simulink model "Modeloplanta"  (R2019a)
settings: Solver=VariableStepAuto  StartTime=0.0  StopTime=10.0  RelTol=1e-3
values from neighbouring files (symbols this model uses):
  A = 2.7    [parámetros.m]
  B = 0.1    [parámetros.m]
  Cr = 0.9    [parámetros.m]
  g = 9.81    [parámetros.m]
  J = 0.002    [parámetros.m]
  K = 0.21    [parámetros.m]
  k = 6.1e-3    (= 0.0061)    [parámetros.m]
  K_bat = (72 / sqrt(3)) / Vdc    [parámetros.m]
  Ki = 7e-1    (= 0.7)    [parámetros.m]
  Kin = 0.6 * (Vdc / Vcm)    [parámetros.m]
  Kp = 105.999    [parámetros.m]
  Kt = sqrt(3) * lamdaf * npp    [parámetros.m]
  L = 86e-6    (= 8.6e-05)    [parámetros.m]
  lamdaf = 0.03    [parámetros.m]
  Loss = 1e-3    (= 0.001)    [parámetros.m]
  Mt = 700    [parámetros.m]
  npp = 16    [parámetros.m]
  Q0 = 3.3 * 72    (= 237.6)    [parámetros.m]
  Qmax = 3.3 * 72    (= 237.6)    [parámetros.m]
  r = 0.049    [parámetros.m]
  rho = 1.3    [parámetros.m]
  RPM_MAX = 800    [parámetros.m]
  rr = 0.3    [parámetros.m]
  Tin = 1 / (2 * fc)    (= 6.25e-05)    [parámetros.m]
  TORQUE_MAX = 140    [parámetros.m]
  Ts = 1e-6    (= 1e-06)    [parámetros.m]
  V = Vdc    (= 106)    [parámetros.m]
  Varnoise = 0    [parámetros.m]
  Vmax = (1/sqrt(3)) * Vdc    [parámetros.m]
  Xnoise = 0    [parámetros.m]
undefined symbols (not defined in the file or in its folder): CARGA
libraries: simulink x1
settings Model: Creator=luisd  LastModifiedBy=luisd

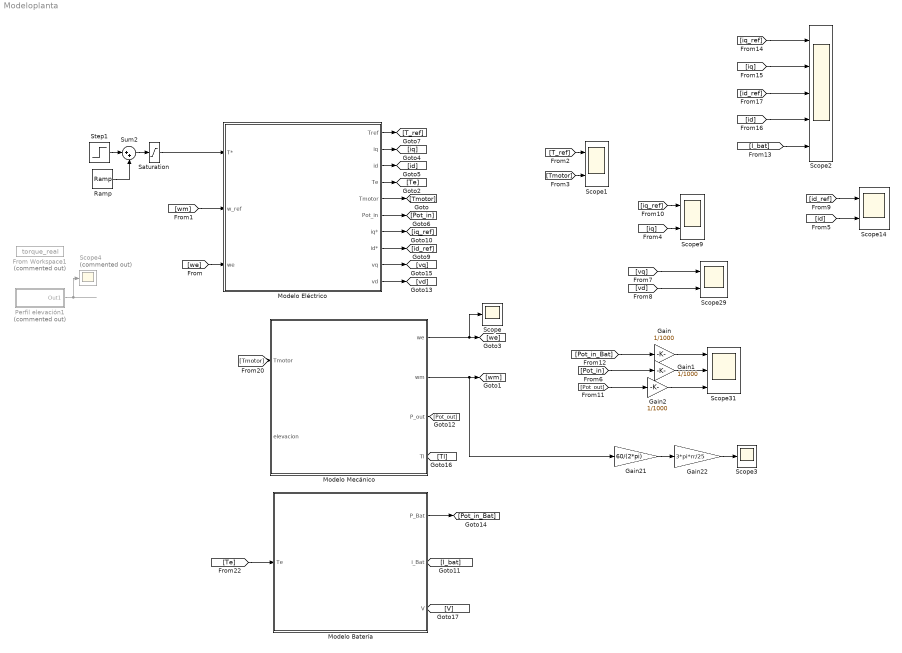
== system Modeloplanta ==
  From Workspace1 : FromWorkspace  Commented=on  VariableName=torque_real
  Gain : Gain  Gain=1/1000
  Gain1 : Gain  Gain=1/1000
  Gain2 : Gain  Gain=1/1000
  Gain21 : Gain  Gain=60/(2*pi)
  Gain22 : Gain  Gain=3*pi*rr/25
  Modelo Batería : Subsystem
  Modelo Eléctrico : Subsystem
      mask Display: image(imread('SEVCON-GEN4-SIZE-42.png'))
  Modelo Mecánico : Subsystem
      mask Display: image(imread('qs.png'))
  Perfil elevación1 : Subsystem  Commented=on
  Ramp : simulink/Sources/Ramp  slope=1e4  start=0.45  InitialOutput=0
  Saturation : Saturate  UpperLimit=5  LowerLimit=0  ZeroCross=off
  Scope : Scope
  Scope{1,9,14,29} (4 alike) : Scope  NumInputPorts=2
  Scope2 : Scope  NumInputPorts=5
  Scope3 : Scope
  Scope31 : Scope  NumInputPorts=3
  Scope4 : Scope  Commented=on
  Step1 : Step  Time=0.5  SampleTime=0
  Sum2 : Sum  Inputs=|++
  wires:
  Gain21/1 -> Gain22/1
  [id] -> Scope2/4
  [vd] -> Scope29/2
  Modelo Eléctrico/3(id) -> [id]
  [iq] -> Scope2/2
  Modelo Eléctrico/5(Tmotor) -> [Tmotor]
  Modelo Eléctrico/1(Tref) -> [T_ref]
  [id_ref] -> Scope2/3
  [I_bat] -> Scope2/5
  [wm] -> Modelo Eléctrico/2(w_ref)
  Modelo Mecánico/3(P_out) -> [Pot_out]
  Gain22/1 -> Scope3/1
  Sum2/1 -> Saturation/1
  Modelo Eléctrico/7(iq*) -> [iq_ref]
  Modelo Mecánico/1(we) -> Scope/1, [we]
  Modelo Eléctrico/8(id*) -> [id_ref]
  Modelo Mecánico/2(wm) -> Gain21/1, [wm]
  Saturation/1 -> Modelo Eléctrico/1(T*)
  [we] -> Modelo Eléctrico/3(we)
  [Pot_in_Bat] -> Gain/1
  Ramp/1 -> Sum2/2
  [vq] -> Scope29/1
  Modelo Batería/1("P_Bat ") -> [Pot_in_Bat]
  [iq_ref] -> Scope9/1
  Modelo Batería/2(i_Bat) -> [I_bat]
  [Tmotor] -> Scope1/2
  Modelo Eléctrico/9(vq) -> [vq]
  Modelo Eléctrico/2(iq) -> [iq]
  [id_ref] -> Scope14/1
  [Pot_out] -> Gain2/1
  Modelo Mecánico/4(Tl) -> [Tl]
  [Pot_in] -> Gain1/1
  Step1/1 -> Sum2/1
  Gain/1 -> Scope31/1
  Modelo Eléctrico/4(Te) -> [Te]
  [Tmotor] -> Modelo Mecánico/1(Tmotor)
  Modelo Eléctrico/10(vd) -> [vd]
  Perfil elevación1/1(Out1) -> Scope4/1
  Gain2/1 -> Scope31/3
  [Te] -> Modelo Batería/1(Te)
  [T_ref] -> Scope1/1
  Modelo Batería/3(V) -> [V]
  [id] -> Scope14/2
  Modelo Eléctrico/6(Pot_in) -> [Pot_in]
  [iq_ref] -> Scope2/1
  [iq] -> Scope9/2
  Gain1/1 -> Scope31/2

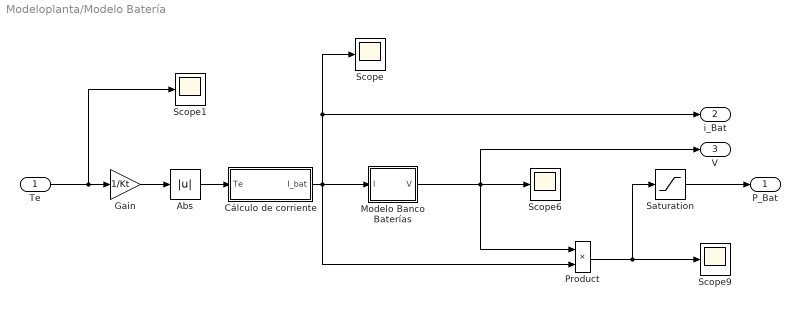
== system Modeloplanta/Modelo Batería ==
  Te : Inport
  Abs : Abs
  Cálculo de corriente : Subsystem
  Gain : Gain  Gain=1/Kt
  Modelo Banco Baterías : Subsystem
  Product : Product
  Saturation : Saturate  UpperLimit=8000  LowerLimit=-8000
  Scope{,1,6,9} (4 alike) : Scope
  "P_Bat " : Outport
  i_Bat : Outport  Port=2
  V : Outport  Port=3
  wires:
  Product/1 -> Saturation/1, Scope9/1
  Modelo Banco Baterías/1(V) -> V/1, Scope6/1, Product/1
  Cálculo de corriente/1(I_bat) -> Scope/1, i_Bat/1, Modelo Banco Baterías/1(I), Product/2
  Te/1 -> Scope1/1, Gain/1
  Saturation/1 -> "P_Bat "/1
  Gain/1 -> Abs/1
  Abs/1 -> Cálculo de corriente/1(Te)

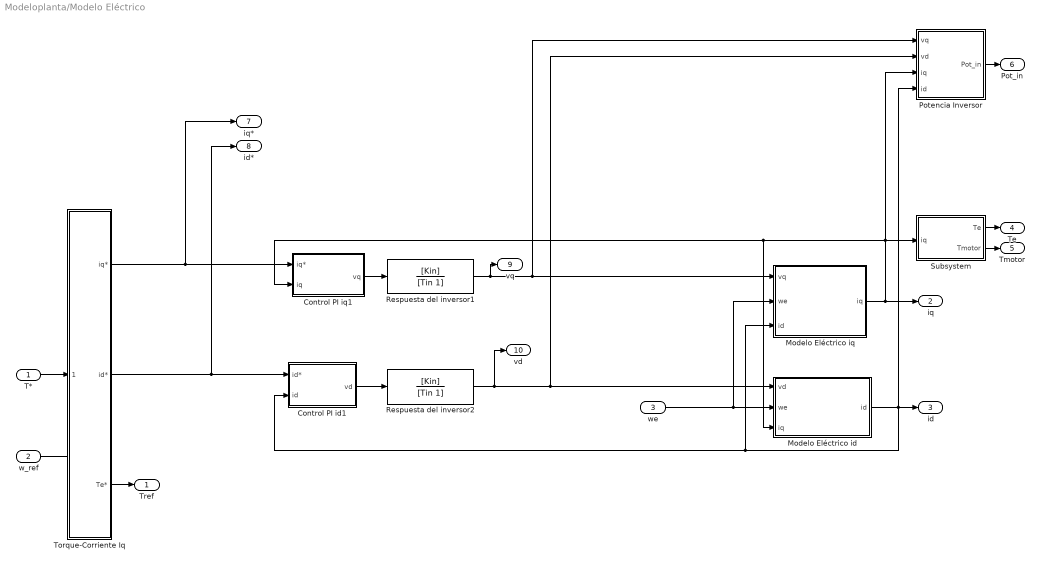
== system Modeloplanta/Modelo Eléctrico ==
  T* : Inport
  w_ref : Inport  Port=2
  we : Inport  Port=3
  Control PI id1 : Subsystem
  Control PI iq1 : Subsystem
  Modelo Eléctrico id : Subsystem
  Modelo Eléctrico iq : Subsystem
  Potencia Inversor : Subsystem
  Respuesta del inversor1 : TransferFcn  Numerator=[Kin]  Denominator=[Tin 1]
  Respuesta del inversor2 : TransferFcn  Numerator=[Kin]  Denominator=[Tin 1]
  Subsystem : Subsystem
  Torque-Corriente Iq : Subsystem
  Tref : Outport
  iq : Outport  Port=2
  id : Outport  Port=3
  Te : Outport  Port=4
  Tmotor : Outport  Port=5
  Pot_in : Outport  Port=6
  iq* : Outport  Port=7
  id* : Outport  Port=8
  vq : Outport  Port=9
  vd : Outport  Port=10
  wires:
  Modelo Eléctrico iq/1(iq) -> iq/1, Control PI iq1/2(iq), Modelo Eléctrico id/3(iq), Subsystem/1(iq), Potencia Inversor/3(iq)
  Subsystem/1(Te) -> Te/1
  Torque-Corriente Iq/2(id*) -> Control PI id1/1(id*), id*/1
  Subsystem/2(Tmotor) -> Tmotor/1
  Torque-Corriente Iq/3(Te*) -> Tref/1
  w_ref/1 -> ?
  T*/1 -> Torque-Corriente Iq/1(Tdmd*)
  Torque-Corriente Iq/1(iq*) -> Control PI iq1/1(iq*), iq*/1
  Potencia Inversor/1(Pot_in) -> Pot_in/1
  we/1 -> Modelo Eléctrico iq/2(we), Modelo Eléctrico id/2(we)
  Modelo Eléctrico id/1(id) -> id/1, Control PI id1/2(id), Modelo Eléctrico iq/3(id), Potencia Inversor/4(id)
  Control PI iq1/1(vq) -> Respuesta del inversor1/1
  Control PI id1/1(vd) -> Respuesta del inversor2/1
  Respuesta del inversor1/1 -> vq/1, Modelo Eléctrico iq/1(vq), Potencia Inversor/1(vq)
  Respuesta del inversor2/1 -> Potencia Inversor/2(vd), Modelo Eléctrico id/1(vd), vd/1

== system Modeloplanta/Modelo Mecánico ==
  Tmotor : Inport
  elevacion : Inport  Port=2
  Modelo Mecánico : Subsystem
  Potencia de Salida : Subsystem
  Scope30 : Scope
  Torque en la carga : Subsystem
  velocidad mecánica a électrica : Subsystem
  we : Outport
  wm : Outport  Port=2
  P_out : Outport  Port=3
  Tl : Outport  Port=4
  wires:
  Tmotor/1 -> Potencia de Salida/1(Tmotor), Modelo Mecánico/1(Tmotor)
  Torque en la carga/1(Tl) -> Tl/1, Modelo Mecánico/2(Tl)
  velocidad mecánica a électrica/1(we) -> we/1
  Potencia de Salida/1(Pout) -> P_out/1
  Modelo Mecánico/1(wm) -> wm/1, Potencia de Salida/2(wm), Torque en la carga/2(wm), velocidad mecánica a électrica/1(wm)
  elevacion/1 -> Torque en la carga/1(alfaº), Scope30/1

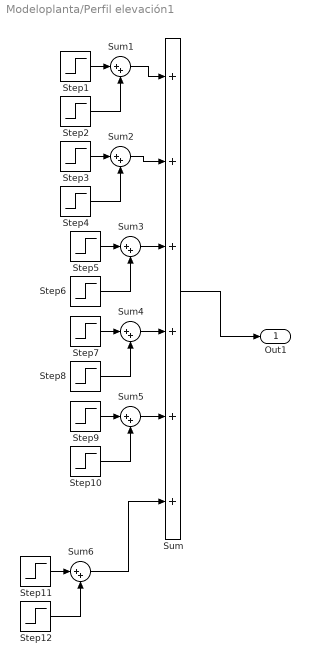
== system Modeloplanta/Perfil elevación1 ==
  Step1 : Step  Time=190  After=-1.5  SampleTime=0
  Step10 : Step  Time=850  After=1.5  SampleTime=0
  Step11 : Step  Time=50  After=-1  SampleTime=0
  Step12 : Step  Time=85  SampleTime=0
  Step2 : Step  Time=235.48  After=1.5  SampleTime=0
  Step3 : Step  Time=330  After=-1.5  SampleTime=0
  Step4 : Step  Time=410  After=1.5  SampleTime=0
  Step5 : Step  Time=490  After=-1.5  SampleTime=0
  Step6 : Step  Time=560  After=1.5  SampleTime=0
  Step7 : Step  Time=640  After=-1.5  SampleTime=0
  Step8 : Step  Time=710  After=1.5  SampleTime=0
  Step9 : Step  Time=790  After=-1.5  SampleTime=0
  Sum : Sum  Inputs=++++++
  Sum{1..6} (6 alike) : Sum  Inputs=|++
  Out1 : Outport
  wires:
  Sum3/1 -> Sum/3
  Sum1/1 -> Sum/1
  Sum4/1 -> Sum/4
  Step7/1 -> Sum4/1
  Step10/1 -> Sum5/2
  Sum/1 -> Out1/1
  Step9/1 -> Sum5/1
  Sum2/1 -> Sum/2
  Step8/1 -> Sum4/2
  Sum5/1 -> Sum/5
  Step6/1 -> Sum3/2
  Sum6/1 -> Sum/6
  Step4/1 -> Sum2/2
  Step3/1 -> Sum2/1
  Step5/1 -> Sum3/1
  Step11/1 -> Sum6/1
  Step12/1 -> Sum6/2
  Step2/1 -> Sum1/2
  Step1/1 -> Sum1/1

== system Modeloplanta/Modelo Batería/Cálculo de corriente ==
  Te : Inport
  Gain1 : Gain  Gain=K_bat
  Saturation : Saturate  UpperLimit=inf  LowerLimit=0  ZeroCross=off
  I_bat : Outport
  wires:
  Gain1/1 -> Saturation/1
  Saturation/1 -> I_bat/1
  Te/1 -> Gain1/1

== system Modeloplanta/Modelo Batería/Modelo Banco Baterías ==
  I : Inport
  "A -> Ah" : Gain  Gain=-1/3600
  Q (Ah) : Integrator  InitialCondition=Q0  LimitOutput=on  UpperSaturationLimit=Qmax  LowerSaturationLimit=0
  Q->SOC : Gain  Gain=1/Qmax
  "SOC -> Voltage" : Subsystem  mask{Vn=V, K_C=K, C_loss=Loss}
      mask prompts: Vn "Constant Voltage (V)"; K_C "Polarization Resistance (ohm)"; C_loss "Charging loss (%)"
  Scope : Scope
  Scope1 : Scope
  V : Outport
  wires:
  "A -> Ah"/1 -> Scope/1, Q (Ah)/1
  Q->SOC/1 -> "SOC -> Voltage"/1(SOC)
  Q (Ah)/1 -> Scope1/1, Q->SOC/1
  "SOC -> Voltage"/1(Voltage) -> V/1
  I/1 -> "SOC -> Voltage"/2(Current), "A -> Ah"/1

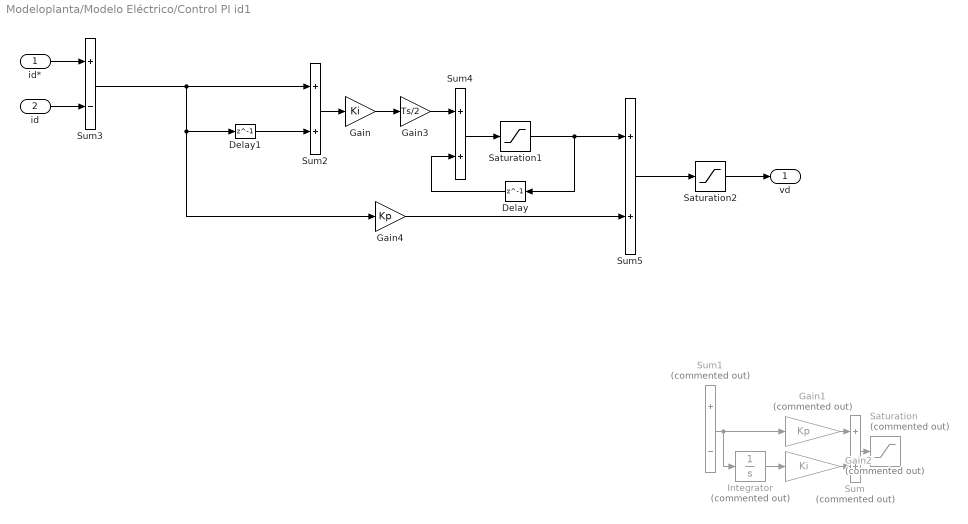
== system Modeloplanta/Modelo Eléctrico/Control PI id1 ==
  id* : Inport
  id : Inport  Port=2
  Delay : Delay  DelayLength=1
  Delay1 : Delay  DelayLength=1
  Gain : Gain  Gain=Ki
  Gain1 : Gain  Commented=on  Gain=Kp
  Gain2 : Gain  Commented=on  Gain=Ki
  Gain3 : Gain  Gain=Ts/2
  Gain4 : Gain  Gain=Kp
  Integrator : Integrator  Commented=on
  Saturation : Saturate  Commented=on  UpperLimit=Vmax  LowerLimit=-Vmax
  Saturation1 : Saturate  UpperLimit=inf  LowerLimit=-inf
  Saturation2 : Saturate  UpperLimit=Vmax  LowerLimit=-Vmax
  Sum : Sum  Commented=on
  Sum1 : Sum  Commented=on  Inputs=+-
  Sum2 : Sum
  Sum3 : Sum  Inputs=+-
  Sum4 : Sum
  Sum5 : Sum
  vd : Outport
  wires:
  Gain2/1 -> Sum/2
  Integrator/1 -> Gain2/1
  Sum1/1 -> Gain1/1, Integrator/1
  Gain1/1 -> Sum/1
  Sum/1 -> Saturation/1
  id/1 -> Sum3/2
  Delay/1 -> Sum4/2
  Sum5/1 -> Saturation2/1
  Sum2/1 -> Gain/1
  id*/1 -> Sum3/1
  Gain3/1 -> Sum4/1
  Sum3/1 -> Sum2/1, Gain4/1, Delay1/1
  Delay1/1 -> Sum2/2
  Sum4/1 -> Saturation1/1
  Saturation1/1 -> Delay/1, Sum5/1
  Gain4/1 -> Sum5/2
  Gain/1 -> Gain3/1
  Saturation2/1 -> vd/1

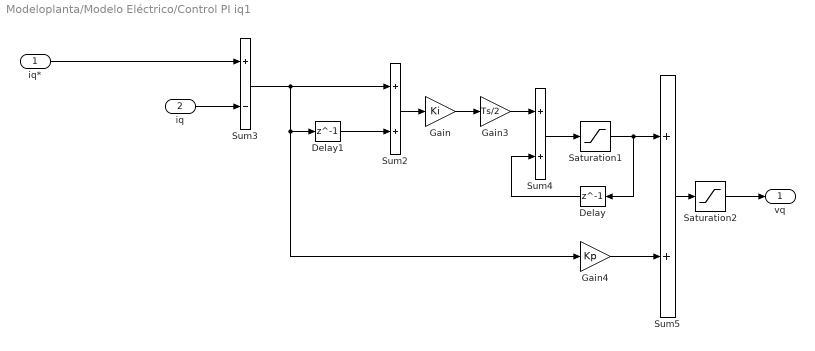
== system Modeloplanta/Modelo Eléctrico/Control PI iq1 ==
  iq* : Inport
  iq : Inport  Port=2
  Delay : Delay  DelayLength=1
  Delay1 : Delay  DelayLength=1
  Gain : Gain  Gain=Ki
  Gain3 : Gain  Gain=Ts/2
  Gain4 : Gain  Gain=Kp
  Saturation1 : Saturate  UpperLimit=inf  LowerLimit=-inf
  Saturation2 : Saturate  UpperLimit=Vmax  LowerLimit=-Vmax
  Sum2 : Sum
  Sum3 : Sum  Inputs=+-
  Sum4 : Sum
  Sum5 : Sum
  vq : Outport
  wires:
  Saturation2/1 -> vq/1
  iq/1 -> Sum3/2
  Delay/1 -> Sum4/2
  Sum5/1 -> Saturation2/1
  Sum2/1 -> Gain/1
  Gain3/1 -> Sum4/1
  Sum3/1 -> Sum2/1, Gain4/1, Delay1/1
  Delay1/1 -> Sum2/2
  Sum4/1 -> Saturation1/1
  Saturation1/1 -> Sum5/1, Delay/1
  Gain4/1 -> Sum5/2
  Gain/1 -> Gain3/1
  iq*/1 -> Sum3/1

== system Modeloplanta/Modelo Eléctrico/Modelo Eléctrico id ==
  vd : Inport
  we : Inport  Port=2
  iq : Inport  Port=3
  Gain : Gain  Gain=1/L
  Gain2 : Gain  Gain=r
  Gain3 : Gain  Gain=L
  Integrator : Integrator
  Product : Product
  Sum : Sum  Inputs=++-
  id : Outport
  wires:
  we/1 -> Product/1
  Sum/1 -> Gain/1
  Product/1 -> Gain3/1
  Gain/1 -> Integrator/1
  Gain3/1 -> Sum/2
  iq/1 -> Product/2
  Gain2/1 -> Sum/3
  Integrator/1 -> id/1, Gain2/1
  vd/1 -> Sum/1

== system Modeloplanta/Modelo Eléctrico/Modelo Eléctrico iq ==
  vq : Inport
  we : Inport  Port=2
  id : Inport  Port=3
  Constant : Constant  Value=lamdaf
  Gain : Gain  Gain=1/L
  Gain1 : Gain  Gain=r
  Gain3 : Gain  Gain=L
  Integrator : Integrator
  Product : Product
  Sum : Sum  Inputs=+--
  Sum1 : Sum
  iq : Outport
  wires:
  Constant/1 -> Sum1/2
  Gain/1 -> Integrator/1
  vq/1 -> Sum/1
  Sum/1 -> Gain/1
  Product/1 -> Sum/2
  Gain3/1 -> Sum1/1
  id/1 -> Gain3/1
  Sum1/1 -> Product/2
  Gain1/1 -> Sum/3
  we/1 -> Product/1
  Integrator/1 -> iq/1, Gain1/1

== system Modeloplanta/Modelo Eléctrico/Potencia Inversor ==
  vq : Inport
  vd : Inport  Port=2
  iq : Inport  Port=3
  id : Inport  Port=4
  Gain1 : Gain  Gain=3/2
  Product : Product
  Product1 : Product
  Scope : Scope
  Scope1 : Scope
  Sum : Sum
  Pot_in : Outport
  wires:
  iq/1 -> Product/1
  id/1 -> Product1/1
  Product/1 -> Sum/1, Scope1/1
  Product1/1 -> Scope/1, Sum/2
  Sum/1 -> Gain1/1
  Gain1/1 -> Pot_in/1
  vq/1 -> Product/2
  vd/1 -> Product1/2

== system Modeloplanta/Modelo Eléctrico/Subsystem ==
  iq : Inport
  Corriente a torque : Subsystem
  Torque motor : Subsystem
  Te : Outport
  Tmotor : Outport  Port=2
  wires:
  Corriente a torque/1("Tmotor ") -> Te/1, Torque motor/1(Te)
  iq/1 -> Corriente a torque/1(Iq)
  Torque motor/1(Tmotor) -> Tmotor/1

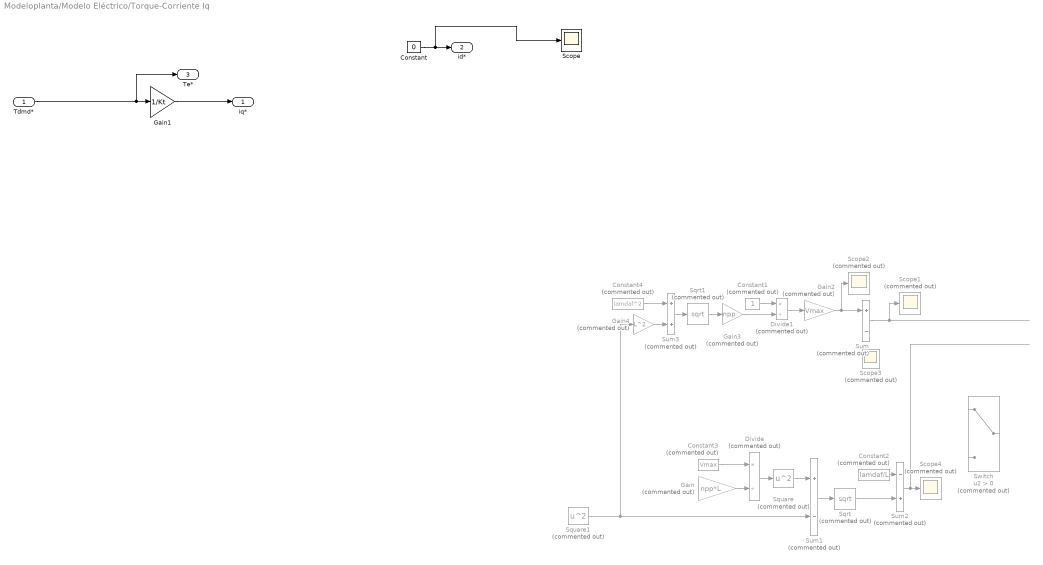
== system Modeloplanta/Modelo Eléctrico/Torque-Corriente Iq ==
  Tdmd* : Inport
  Constant : Constant  Value=0
  Constant1 : Constant  Commented=on
  Constant2 : Constant  Commented=on  Value=lamdaf/L
  Constant3 : Constant  Commented=on  Value=Vmax
  Constant4 : Constant  Commented=on  Value=lamdaf^2
  Divide : Product  Commented=on  Inputs=*/
  Divide1 : Product  Commented=on  Inputs=*/
  Gain : Gain  Commented=on  Gain=npp*L
  Gain1 : Gain  Gain=1/Kt
  Gain2 : Gain  Commented=on  Gain=Vmax
  Gain3 : Gain  Commented=on  Gain=npp
  Gain4 : Gain  Commented=on  Gain=L^2
  Scope : Scope
  Scope{1..4} (4 alike) : Scope  Commented=on
  Sqrt : Sqrt  Commented=on  SaturateOnIntegerOverflow=on
  Sqrt1 : Sqrt  Commented=on  SaturateOnIntegerOverflow=on
  Square : Math  Commented=on  Operator=square  SaturateOnIntegerOverflow=on
  Square1 : Math  Commented=on  Operator=square  SaturateOnIntegerOverflow=on
  Sum : Sum  Commented=on  Inputs=+-
  Sum1 : Sum  Commented=on  Inputs=+-
  Sum2 : Sum  Commented=on  Inputs=-+
  Sum3 : Sum  Commented=on
  Switch : Switch  Commented=on  Criteria=u2 > Threshold
  iq* : Outport
  id* : Outport  Port=2
  Te* : Outport  Port=3
  wires:
  Constant/1 -> Scope/1, id*/1
  Gain1/1 -> iq*/1
  Tdmd*/1 -> Te*/1, Gain1/1
  Sum2/1 -> Scope4/1
  Sqrt/1 -> Sum2/2
  Sum/1 -> Scope1/1
  Gain3/1 -> Divide1/2
  Constant4/1 -> Sum3/1
  Gain/1 -> Divide/2
  Sum1/1 -> Sqrt/1
  Constant1/1 -> Divide1/1
  Gain4/1 -> Sum3/2
  Divide/1 -> Square/1
  Sqrt1/1 -> Gain3/1
  Sum3/1 -> Sqrt1/1
  Divide1/1 -> Gain2/1
  Constant3/1 -> Divide/1
  Square/1 -> Sum1/1
  Gain2/1 -> Sum/1, Scope2/1
  Constant2/1 -> Sum2/1
  ? -> Gain/1, Scope3/1, Sum/2
  Square1/1 -> Gain4/1, Sum1/2

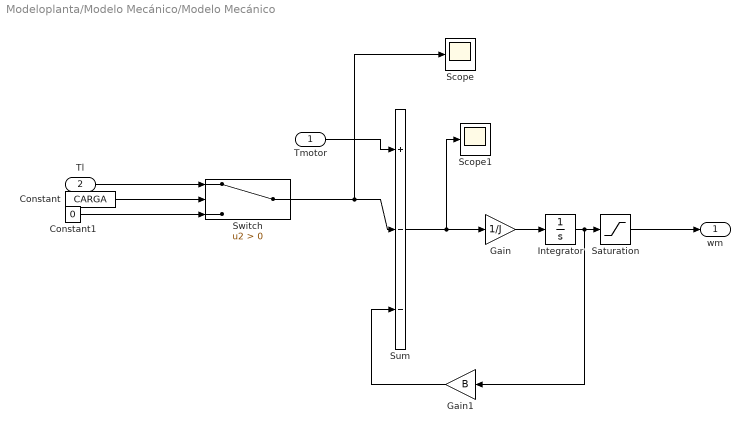
== system Modeloplanta/Modelo Mecánico/Modelo Mecánico ==
  Tmotor : Inport
  Tl : Inport  Port=2
  Constant : Constant  Value=CARGA
  Constant1 : Constant  Value=0
  Gain : Gain  Gain=1/J
  Gain1 : Gain  Gain=B
  Integrator : Integrator
  Saturation : Saturate  UpperLimit=(2*pi*RPM_MAX)/60  LowerLimit=-(2*pi*RPM_MAX)/60  ZeroCross=off
  Scope : Scope
  Scope1 : Scope
  Sum : Sum  Inputs=+--
  Switch : Switch  Criteria=u2 > Threshold
  wm : Outport
  wires:
  Gain/1 -> Integrator/1
  Tmotor/1 -> Sum/1
  Integrator/1 -> Gain1/1, Saturation/1
  Switch/1 -> Scope/1, Sum/2
  Constant1/1 -> Switch/3
  Constant/1 -> Switch/2
  Tl/1 -> Switch/1
  Saturation/1 -> wm/1
  Gain1/1 -> Sum/3
  Sum/1 -> Scope1/1, Gain/1

== system Modeloplanta/Modelo Mecánico/Potencia de Salida ==
  Tmotor : Inport
  wm : Inport  Port=2
  Product : Product
  Saturation : Saturate  UpperLimit=4000  LowerLimit=-4000
  Scope8 : Scope
  Pout : Outport
  wires:
  Product/1 -> Saturation/1
  wm/1 -> Product/2, Scope8/1
  Tmotor/1 -> Product/1
  Saturation/1 -> Pout/1

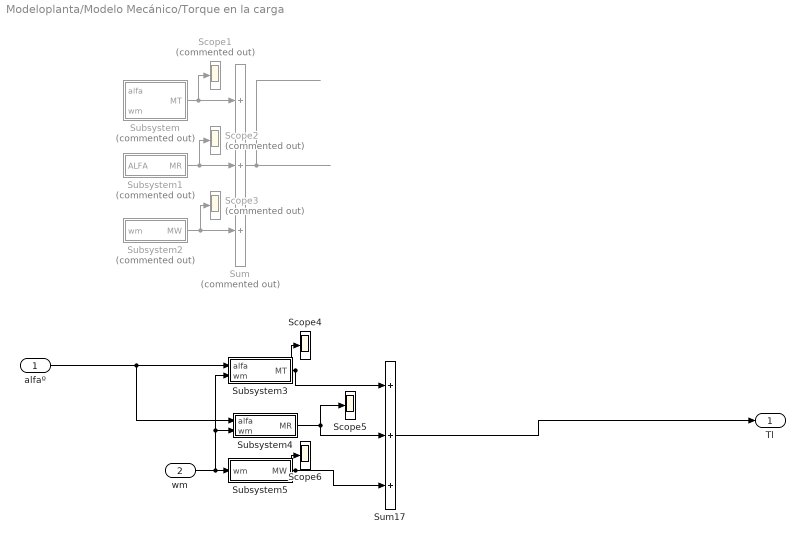
== system Modeloplanta/Modelo Mecánico/Torque en la carga ==
  alfaº : Inport
  wm : Inport  Port=2
  Scope1 : Scope  Commented=on
  Scope2 : Scope  Commented=on
  Scope3 : Scope  Commented=on
  Scope4 : Scope
  Scope5 : Scope
  Scope6 : Scope
  Subsystem : Subsystem  Commented=on
  Subsystem1 : Subsystem  Commented=on
  Subsystem2 : Subsystem  Commented=on
  Subsystem3 : Subsystem
  Subsystem4 : Subsystem
  Subsystem5 : Subsystem
  Sum : Sum  Commented=on  Inputs=+++
  Sum17 : Sum  Inputs=+++
  Tl : Outport
  wires:
  Sum/1 -> ?
  Subsystem/1(MT) -> Scope1/1, Sum/1
  Subsystem1/1(MR) -> Scope2/1, Sum/2
  Subsystem2/1(MW) -> Scope3/1, Sum/3
  Subsystem5/1(MW) -> Scope6/1, Sum17/3
  alfaº/1 -> Subsystem3/1(alfa), Subsystem4/1(alfa)
  Sum17/1 -> Tl/1
  wm/1 -> Subsystem5/1(wm), Subsystem3/2(wm), Subsystem4/2(wm)
  Subsystem4/1(MR) -> Scope5/1, Sum17/2
  Subsystem3/1(MT) -> Scope4/1, Sum17/1

== system Modeloplanta/Modelo Mecánico/velocidad mecánica a électrica ==
  wm : Inport
  Gain : Gain  Gain=npp
  we : Outport
  wires:
  wm/1 -> Gain/1
  Gain/1 -> we/1

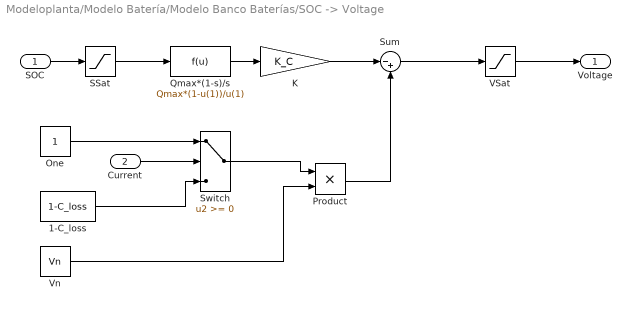
== system Modeloplanta/Modelo Batería/Modelo Banco Baterías/SOC -> Voltage ==
  SOC : Inport
  Current : Inport  Port=2
  1-C_loss : Constant  Value=1-C_loss
  K : Gain  Gain=K_C
  One : Constant
  Product : Product  RndMeth=Zero
  Qmax*(1-s)/s : Fcn  Expr=Qmax*(1-u(1))/u(1)
  SSat : Saturate  UpperLimit=1  LowerLimit=eps
  Sum : Sum  Inputs=|-+
  Switch : Switch
  VSat : Saturate  UpperLimit=inf  LowerLimit=0
  Vn : Constant  Value=Vn
  Voltage : Outport
  wires:
  1-C_loss/1 -> Switch/3
  SOC/1 -> SSat/1
  Current/1 -> Switch/2
  Qmax*(1-s)/s/1 -> K/1
  One/1 -> Switch/1
  VSat/1 -> Voltage/1
  K/1 -> Sum/1
  Switch/1 -> Product/1
  Vn/1 -> Product/2
  Product/1 -> Sum/2
  Sum/1 -> VSat/1
  SSat/1 -> Qmax*(1-s)/s/1

== system Modeloplanta/Modelo Eléctrico/Subsystem/Corriente a torque ==
  Iq : Inport
  Gain1 : Gain  Gain=Kt
  Saturation1 : Saturate  UpperLimit=TORQUE_MAX  LowerLimit=-TORQUE_MAX
  "Tmotor " : Outport
  wires:
  Gain1/1 -> Saturation1/1
  Iq/1 -> Gain1/1
  Saturation1/1 -> "Tmotor "/1

== system Modeloplanta/Modelo Eléctrico/Subsystem/Torque motor ==
  Te : Inport
  Random Number : RandomNumber  Mean=Xnoise  Variance=Varnoise  SampleTime=0.01
  Saturation1 : Saturate  UpperLimit=TORQUE_MAX  LowerLimit=-TORQUE_MAX
  Scope : Scope
  Scope6 : Scope
  Sum2 : Sum
  Tmotor : Outport
  wires:
  Sum2/1 -> Scope6/1, Saturation1/1
  Random Number/1 -> Scope/1, Sum2/2
  Te/1 -> Sum2/1
  Saturation1/1 -> Tmotor/1

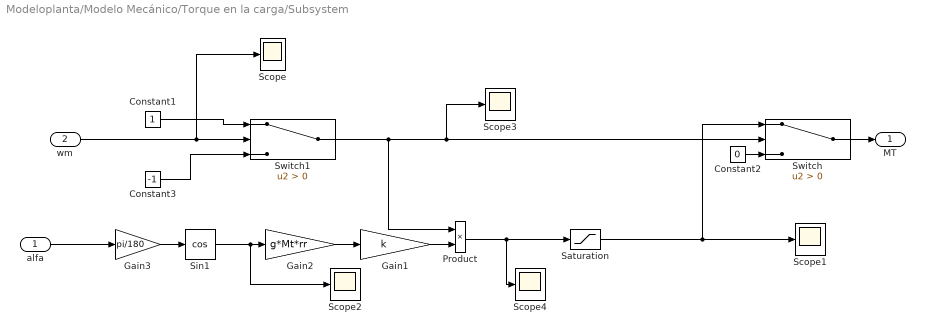
== system Modeloplanta/Modelo Mecánico/Torque en la carga/Subsystem ==
  alfa : Inport
  wm : Inport  Port=2
  Constant1 : Constant
  Constant2 : Constant  Value=0
  Constant3 : Constant  Value=-1
  Gain1 : Gain  Gain=k
  Gain2 : Gain  Gain=g*Mt*rr
  Gain3 : Gain  Gain=pi/180
  Product : Product
  Saturation : Saturate  UpperLimit=inf  LowerLimit=0  ZeroCross=off
  Scope{,1..4} (5 alike) : Scope
  Sin1 : Trigonometry  Operator=cos
  Switch : Switch  Criteria=u2 > Threshold  ZeroCross=off
  Switch1 : Switch  Criteria=u2 > Threshold  ZeroCross=off
  MT : Outport
  wires:
  Sin1/1 -> Scope2/1, Gain2/1
  Gain3/1 -> Sin1/1
  alfa/1 -> Gain3/1
  Gain2/1 -> Gain1/1
  Constant2/1 -> Switch/3
  Switch/1 -> MT/1
  Saturation/1 -> Switch/1, Scope1/1
  Product/1 -> Scope4/1, Saturation/1
  Switch1/1 -> Product/1, Scope3/1, Switch/2
  wm/1 -> Switch1/2, Scope/1
  Constant1/1 -> Switch1/1
  Constant3/1 -> Switch1/3
  Gain1/1 -> Product/2

== system Modeloplanta/Modelo Mecánico/Torque en la carga/Subsystem1 ==
  ALFA : Inport
  Gain1 : Gain  Gain=g*Mt*rr
  Gain5 : Gain  Gain=pi/180
  Scope11 : Scope
  Sin : Trigonometry
  MR : Outport
  wires:
  Gain5/1 -> Sin/1
  Gain1/1 -> Scope11/1, MR/1
  Sin/1 -> Gain1/1
  ALFA/1 -> Gain5/1

== system Modeloplanta/Modelo Mecánico/Torque en la carga/Subsystem2 ==
  wm : Inport
  Gain : Gain  Gain=rr
  Gain6 : Gain  Gain=0.5*Cr*A*rho*rr
  Scope13 : Scope
  Square : Math  Operator=square  SaturateOnIntegerOverflow=on
  MW : Outport
  wires:
  Gain6/1 -> MW/1, Scope13/1
  Square/1 -> Gain6/1
  Gain/1 -> Square/1
  wm/1 -> Gain/1

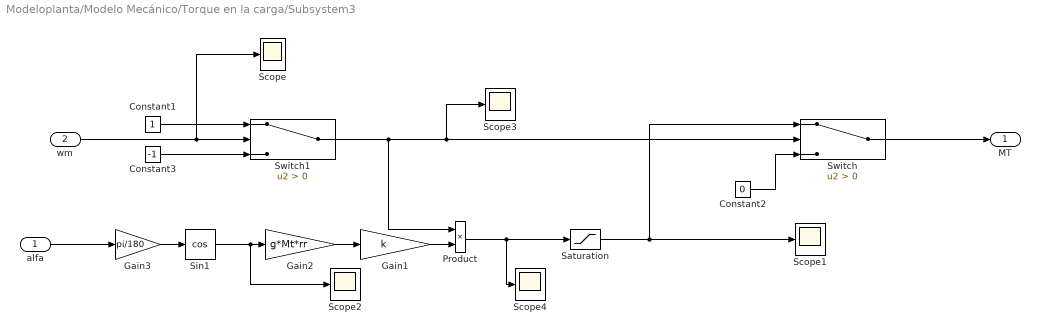
== system Modeloplanta/Modelo Mecánico/Torque en la carga/Subsystem3 ==
  alfa : Inport
  wm : Inport  Port=2
  Constant1 : Constant
  Constant2 : Constant  Value=0
  Constant3 : Constant  Value=-1
  Gain1 : Gain  Gain=k
  Gain2 : Gain  Gain=g*Mt*rr
  Gain3 : Gain  Gain=pi/180
  Product : Product
  Saturation : Saturate  UpperLimit=inf  LowerLimit=-inf  ZeroCross=off
  Scope{,1..4} (5 alike) : Scope
  Sin1 : Trigonometry  Operator=cos
  Switch : Switch  Criteria=u2 > Threshold  ZeroCross=off
  Switch1 : Switch  Criteria=u2 > Threshold  ZeroCross=off
  MT : Outport
  wires:
  Sin1/1 -> Scope2/1, Gain2/1
  Gain3/1 -> Sin1/1
  alfa/1 -> Gain3/1
  Gain2/1 -> Gain1/1
  Constant2/1 -> Switch/3
  Saturation/1 -> Scope1/1, Switch/1
  Product/1 -> Scope4/1, Saturation/1
  wm/1 -> Switch1/2, Scope/1
  Constant1/1 -> Switch1/1
  Constant3/1 -> Switch1/3
  Gain1/1 -> Product/2
  Switch/1 -> MT/1
  Switch1/1 -> Product/1, Switch/2, Scope3/1

== system Modeloplanta/Modelo Mecánico/Torque en la carga/Subsystem4 ==
  alfa : Inport
  wm : Inport  Port=2
  Constant1 : Constant
  Constant3 : Constant  Value=-1
  Gain1 : Gain  Gain=g*Mt*rr
  Gain5 : Gain  Gain=pi/180
  Product : Product
  Scope : Scope
  Scope11 : Scope
  Sin : Trigonometry
  Switch1 : Switch  Criteria=u2 > Threshold  ZeroCross=off
  MR : Outport
  wires:
  Gain5/1 -> Sin/1
  Gain1/1 -> Product/2, Scope11/1
  Sin/1 -> Gain1/1
  alfa/1 -> Gain5/1
  Product/1 -> MR/1
  Constant1/1 -> Switch1/1
  wm/1 -> Switch1/2, Scope/1
  Constant3/1 -> Switch1/3
  Switch1/1 -> Product/1

== system Modeloplanta/Modelo Mecánico/Torque en la carga/Subsystem5 ==
  wm : Inport
  Constant1 : Constant
  Constant3 : Constant  Value=-1
  Gain : Gain  Gain=rr
  Gain6 : Gain  Gain=0.5*Cr*A*rho*rr
  Product : Product
  Scope : Scope
  Scope1 : Scope
  Scope13 : Scope
  Square : Math  Operator=square  SaturateOnIntegerOverflow=on
  Switch1 : Switch  Criteria=u2 > Threshold  ZeroCross=off
  MW : Outport
  wires:
  Square/1 -> Gain6/1
  Gain/1 -> Square/1
  Gain6/1 -> Product/2, Scope13/1
  Constant1/1 -> Switch1/1
  Switch1/1 -> Product/1
  wm/1 -> Scope/1, Switch1/2, Gain/1
  Constant3/1 -> Switch1/3
  Product/1 -> MW/1, Scope1/1
